simulink model "distances"  (R2018b)
settings: Solver=VariableStepAuto  StartTime=0.0  StopTime=1000  RelTol=1e-3
settings Model: Creator=User  LastModifiedBy=User

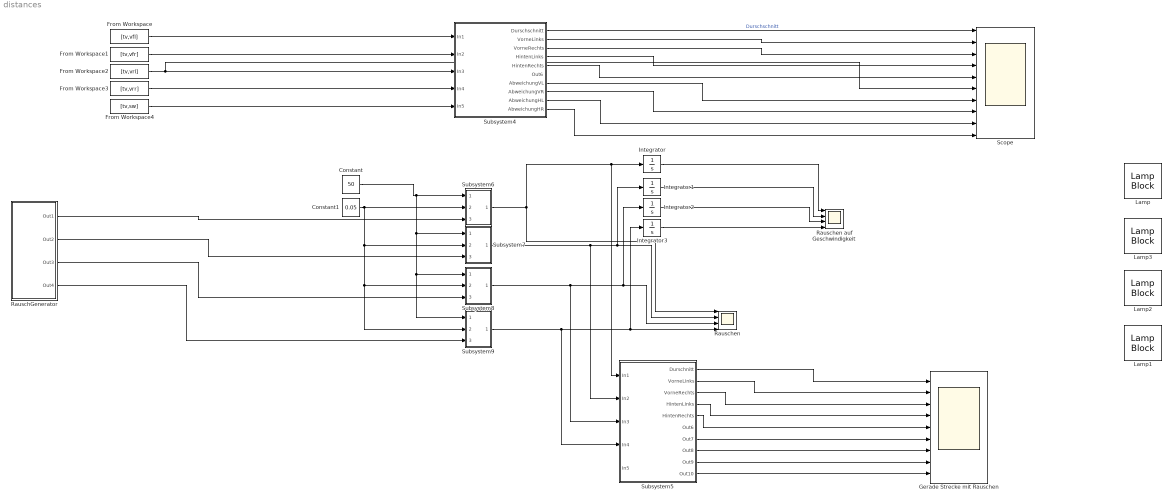
== system distances ==
  Constant : Constant  Value=50
  Constant1 : Constant  Value=0.05
  From Workspace : FromWorkspace  VariableName=[tv,vfl]
  From Workspace1 : FromWorkspace  VariableName=[tv,vfr]
  From Workspace2 : FromWorkspace  VariableName=[tv,vrl]
  From Workspace3 : FromWorkspace  VariableName=[tv,vrr]
  From Workspace4 : FromWorkspace  VariableName=[tv,sw]
  "Gerade Strecke mit Rauschen " : Scope  NumInputPorts=9
  Integrator{,1..3} (4 alike) : Integrator
  Lamp : LampBlock  WebBlockId=126
  Lamp1 : LampBlock  WebBlockId=127
  Lamp2 : LampBlock  WebBlockId=128
  Lamp3 : LampBlock  WebBlockId=129
  RauschGenerator : Subsystem
  "Rauschen " : Scope  NumInputPorts=4
  "Rauschen auf Geschwindigkeit " : Scope  NumInputPorts=4
  Scope : Scope  NumInputPorts=10
  Subsystem4 : Subsystem
  Subsystem5 : Subsystem
  Subsystem6 : Subsystem
  Subsystem7 : Subsystem
  Subsystem8 : Subsystem
  Subsystem9 : Subsystem
  wires:
  From Workspace2/1 -> Subsystem4/3(In3), Scope/6
  From Workspace/1 -> Subsystem4/1(In1)
  From Workspace1/1 -> Subsystem4/2(In2)
  From Workspace3/1 -> Subsystem4/4(In4)
  From Workspace4/1 -> Subsystem4/5(In5)
  Subsystem4/1("Durschschnitt ") -> Scope/1  "Durschschnitt"
  Subsystem4/2(VorneLinks) -> Scope/2
  Subsystem4/3(VorneRechts) -> Scope/3
  Subsystem4/4(HintenLinks) -> Scope/4
  Subsystem4/5(HintenRechts) -> Scope/5
  Subsystem4/7(AbweichungVL) -> Scope/7
  Subsystem4/8(AbweichungVR) -> Scope/8
  Subsystem4/9(AbweichungHL) -> Scope/9
  Subsystem4/10("AbweichungHR ") -> Scope/10
  Subsystem5/2(VorneLinks) -> "Gerade Strecke mit Rauschen "/2
  Constant/1 -> Subsystem9/1(In1), Subsystem8/1(In1), Subsystem7/1(In1), Subsystem6/1(In1)
  Constant1/1 -> Subsystem9/2(In2), Subsystem8/2(In2), Subsystem7/2(In2), Subsystem6/2(In2)
  Subsystem6/1(Out1) -> "Rauschen "/1, Integrator/1, Subsystem5/1(In1)
  Subsystem7/1(Out1) -> "Rauschen "/2, Integrator1/1, Subsystem5/2(In2)
  Subsystem5/3(VorneRechts) -> "Gerade Strecke mit Rauschen "/3
  Subsystem5/4(HintenLinks) -> "Gerade Strecke mit Rauschen "/4
  Subsystem5/5(HintenRechts) -> "Gerade Strecke mit Rauschen "/5
  Integrator/1 -> "Rauschen auf Geschwindigkeit "/1
  Integrator1/1 -> "Rauschen auf Geschwindigkeit "/2
  Subsystem8/1(Out1) -> "Rauschen "/3, Integrator2/1, Subsystem5/3(In3)
  Integrator2/1 -> "Rauschen auf Geschwindigkeit "/3
  Integrator3/1 -> "Rauschen auf Geschwindigkeit "/4
  Subsystem9/1(Out1) -> "Rauschen "/4, Integrator3/1, Subsystem5/4(In4)
  RauschGenerator/1(Out1) -> Subsystem6/3(In3)
  RauschGenerator/2(Out2) -> Subsystem7/3(In3)
  RauschGenerator/3(Out3) -> Subsystem8/3(In3)
  RauschGenerator/4(Out4) -> Subsystem9/3(In3)
  Subsystem5/1(Durschnitt) -> "Gerade Strecke mit Rauschen "/1
  Subsystem5/7(Out7) -> "Gerade Strecke mit Rauschen "/6
  Subsystem5/8(Out8) -> "Gerade Strecke mit Rauschen "/7
  Subsystem5/9(Out9) -> "Gerade Strecke mit Rauschen "/8
  Subsystem5/10(Out10) -> "Gerade Strecke mit Rauschen "/9

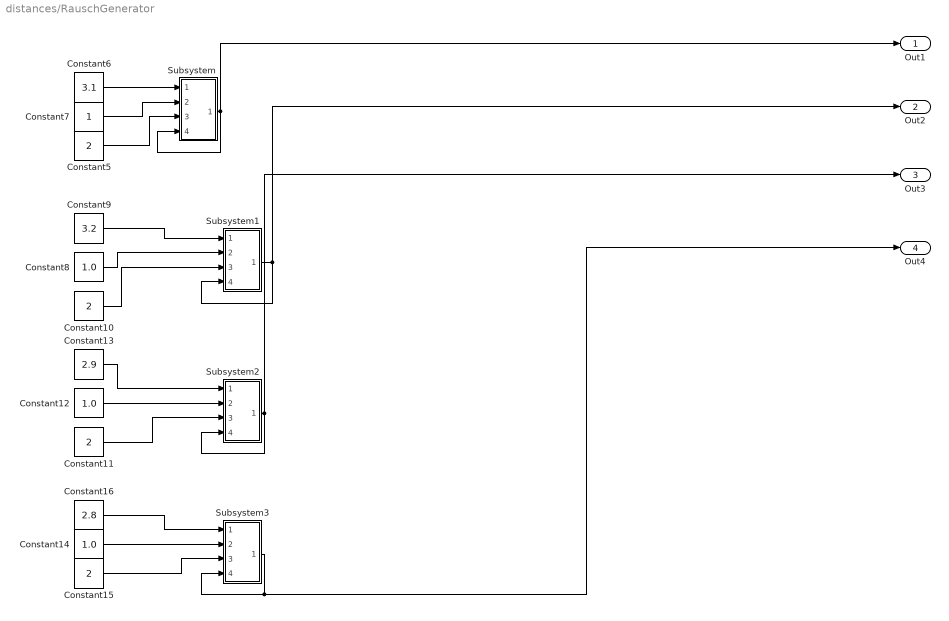
== system distances/RauschGenerator ==
  Constant{5,10..11,15} (4 alike) : Constant  Value=2
  Constant12 : Constant  Value=1.0
  Constant13 : Constant  Value=2.9
  Constant14 : Constant  Value=1.0
  Constant16 : Constant  Value=2.8
  Constant6 : Constant  Value=3.1
  Constant7 : Constant
  Constant8 : Constant  Value=1.0
  Constant9 : Constant  Value=3.2
  Subsystem : Subsystem
  Subsystem1 : Subsystem
  Subsystem2 : Subsystem
  Subsystem3 : Subsystem
  Out1 : Outport
  Out2 : Outport  Port=2
  Out3 : Outport  Port=3
  Out4 : Outport  Port=4
  wires:
  Constant16/1 -> Subsystem3/1(In1)
  Subsystem/1(Out1) -> Out1/1, Subsystem/4(In4)
  Constant11/1 -> Subsystem2/3(In3)
  Constant6/1 -> Subsystem/1(In1)
  Subsystem1/1(Out2) -> Out2/1, Subsystem1/4(In4)
  Subsystem3/1(Out1) -> Out4/1, Subsystem3/4(In4)
  Constant12/1 -> Subsystem2/2(In2)
  Constant5/1 -> Subsystem/3(In3)
  Subsystem2/1(Out1) -> Subsystem2/4(In4), Out3/1
  Constant10/1 -> Subsystem1/3(In3)
  Constant8/1 -> Subsystem1/2(In2)
  Constant9/1 -> Subsystem1/1(In1)
  Constant13/1 -> Subsystem2/1(In1)
  Constant15/1 -> Subsystem3/3(In3)
  Constant14/1 -> Subsystem3/2(In2)
  Constant7/1 -> Subsystem/2(In2)

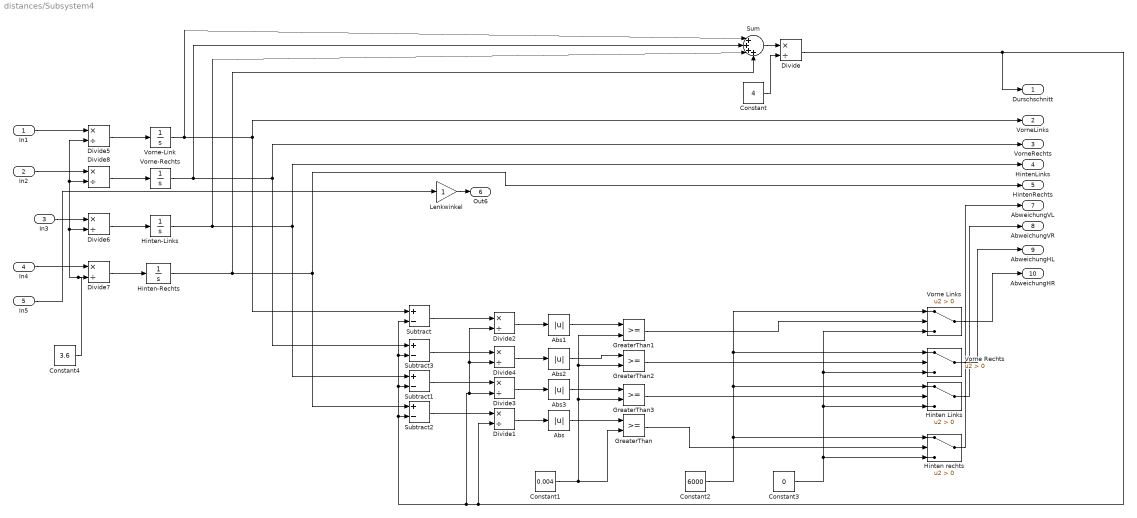
== system distances/Subsystem4 ==
  In1 : Inport
  In2 : Inport  Port=2
  In3 : Inport  Port=3
  In4 : Inport  Port=4
  In5 : Inport  Port=5
  Abs : Abs
  Abs1 : Abs  ZeroCross=off
  Abs2 : Abs
  Abs3 : Abs
  Constant : Constant  Value=4
  Constant1 : Constant  Value=0.004
  Constant2 : Constant  Value=6000
  Constant3 : Constant  Value=0
  Constant4 : Constant  Value=3.6
  Divide{,1..8} (9 alike) : Product  Inputs=*/
  GreaterThan{,1..3} (4 alike) : RelationalOperator  OutDataTypeStr=boolean  RndMeth=Simplest
  Hinten Links : Switch  Criteria=u2 > Threshold
  "Hinten rechts " : Switch  Criteria=u2 > Threshold
  Hinten-Links : Integrator  ContinuousStateAttributes='vfl'
  Hinten-Rechts : Integrator  ContinuousStateAttributes='vfl'
  Lenkwinkel : Gain
  Subtract{,1..3} (4 alike) : Sum  Inputs=+-
  Sum : Sum  Inputs=|++++
  "Vorne Links " : Switch  Criteria=u2 > Threshold
  "Vorne Rechts " : Switch  Criteria=u2 > Threshold
  Vorne-Link : Integrator  ContinuousStateAttributes='vfl'
  Vorne-Rechts : Integrator  ContinuousStateAttributes='vfl'
  "Durschschnitt " : Outport
  VorneLinks : Outport  Port=2
  VorneRechts : Outport  Port=3
  HintenLinks : Outport  Port=4
  HintenRechts : Outport  Port=5
  Out6 : Outport  Port=6
  AbweichungVL : Outport  Port=7
  AbweichungVR : Outport  Port=8
  AbweichungHL : Outport  Port=9
  "AbweichungHR " : Outport  Port=10
  wires:
  Divide5/1 -> Vorne-Link/1
  Divide/1 -> "Durschschnitt "/1, Subtract1/2, Subtract3/2, Subtract/2, Subtract2/2, Divide2/2, Divide4/2, Divide3/2, Divide1/2
  Vorne-Rechts/1 -> VorneRechts/1, Subtract3/1, Sum/2
  Constant4/1 -> Divide6/2, Divide8/2, Divide5/2, Divide7/2
  Abs2/1 -> GreaterThan2/1
  Constant/1 -> Divide/2
  Divide2/1 -> Abs1/1
  Constant3/1 -> "Vorne Links "/3, "Vorne Rechts "/3, Hinten Links/3, "Hinten rechts "/3
  Vorne-Link/1 -> Sum/1, VorneLinks/1, Subtract/1
  Constant2/1 -> "Vorne Links "/1, "Vorne Rechts "/1, Hinten Links/1, "Hinten rechts "/1
  GreaterThan/1 -> "Hinten rechts "/2
  Divide8/1 -> Vorne-Rechts/1
  Divide1/1 -> Abs/1
  Subtract2/1 -> Divide1/1
  Hinten-Links/1 -> HintenLinks/1, Subtract1/1, Sum/3
  Constant1/1 -> GreaterThan/2, GreaterThan3/2, GreaterThan2/2, GreaterThan1/2
  Divide6/1 -> Hinten-Links/1
  In1/1 -> Divide5/1
  Sum/1 -> Divide/1
  Abs3/1 -> GreaterThan3/1
  Abs1/1 -> GreaterThan1/1
  Hinten-Rechts/1 -> HintenRechts/1, Subtract2/1, Sum/4
  Subtract1/1 -> Divide3/1
  Divide4/1 -> Abs2/1
  GreaterThan1/1 -> "Vorne Links "/2
  Subtract/1 -> Divide2/1
  Abs/1 -> GreaterThan/1
  "Vorne Links "/1 -> "AbweichungHR "/1
  GreaterThan2/1 -> "Vorne Rechts "/2
  Subtract3/1 -> Divide4/1
  Divide7/1 -> Hinten-Rechts/1
  Divide3/1 -> Abs3/1
  GreaterThan3/1 -> Hinten Links/2
  "Hinten rechts "/1 -> AbweichungVL/1
  In2/1 -> Divide8/1
  "Vorne Rechts "/1 -> AbweichungHL/1
  In3/1 -> Divide6/1
  Hinten Links/1 -> AbweichungVR/1
  In5/1 -> Lenkwinkel/1
  Lenkwinkel/1 -> Out6/1
  In4/1 -> Divide7/1

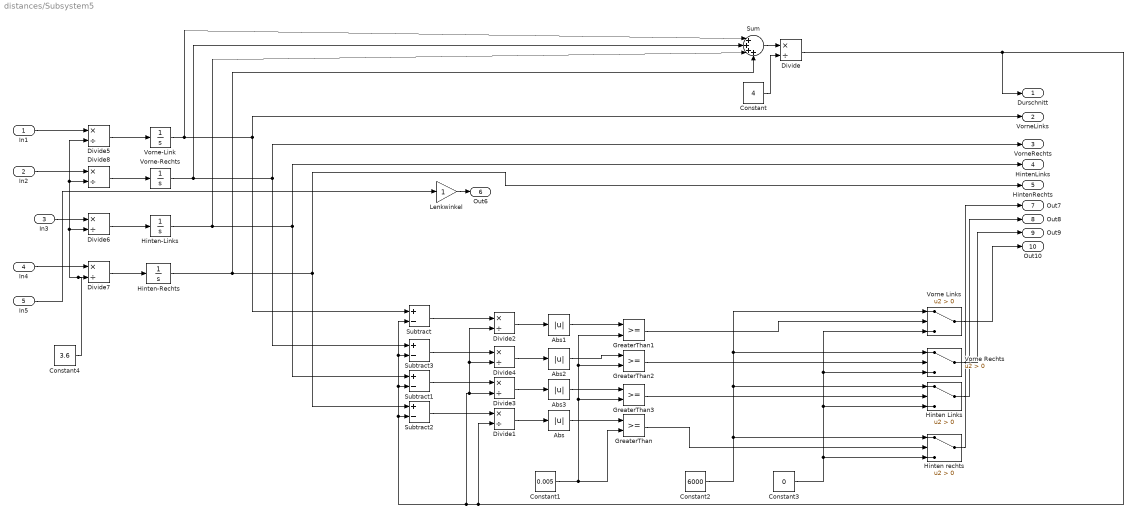
== system distances/Subsystem5 ==
  In1 : Inport
  In2 : Inport  Port=2
  In3 : Inport  Port=3
  In4 : Inport  Port=4
  In5 : Inport  Port=5
  Abs{,1..3} (4 alike) : Abs  ZeroCross=off
  Constant : Constant  Value=4
  Constant1 : Constant  Value=0.005
  Constant2 : Constant  Value=6000
  Constant3 : Constant  Value=0
  Constant4 : Constant  Value=3.6
  Divide{,1..8} (9 alike) : Product  Inputs=*/
  GreaterThan{,1..3} (4 alike) : RelationalOperator  OutDataTypeStr=boolean  ZeroCross=off  RndMeth=Simplest
  Hinten Links : Switch  Criteria=u2 > Threshold
  "Hinten rechts " : Switch  Criteria=u2 > Threshold
  Hinten-Links : Integrator  ContinuousStateAttributes='vfl'
  Hinten-Rechts : Integrator  ContinuousStateAttributes='vfl'
  Lenkwinkel : Gain
  Subtract{,1..3} (4 alike) : Sum  Inputs=+-
  Sum : Sum  Inputs=|++++
  "Vorne Links " : Switch  Criteria=u2 > Threshold
  "Vorne Rechts " : Switch  Criteria=u2 > Threshold
  Vorne-Link : Integrator  ContinuousStateAttributes='vfl'
  Vorne-Rechts : Integrator  ContinuousStateAttributes='vfl'
  Durschnitt : Outport
  VorneLinks : Outport  Port=2
  VorneRechts : Outport  Port=3
  HintenLinks : Outport  Port=4
  HintenRechts : Outport  Port=5
  Out6 : Outport  Port=6
  Out7 : Outport  Port=7
  Out8 : Outport  Port=8
  Out9 : Outport  Port=9
  Out10 : Outport  Port=10
  wires:
  Divide5/1 -> Vorne-Link/1
  Divide/1 -> Durschnitt/1, Subtract1/2, Subtract3/2, Subtract/2, Subtract2/2, Divide2/2, Divide4/2, Divide3/2, Divide1/2
  Vorne-Rechts/1 -> VorneRechts/1, Subtract3/1, Sum/2
  Constant4/1 -> Divide6/2, Divide8/2, Divide5/2, Divide7/2
  Abs2/1 -> GreaterThan2/1
  Constant/1 -> Divide/2
  Divide2/1 -> Abs1/1
  Constant3/1 -> "Vorne Links "/3, "Vorne Rechts "/3, Hinten Links/3, "Hinten rechts "/3
  Vorne-Link/1 -> Sum/1, VorneLinks/1, Subtract/1
  Constant2/1 -> "Vorne Links "/1, "Vorne Rechts "/1, Hinten Links/1, "Hinten rechts "/1
  GreaterThan/1 -> "Hinten rechts "/2
  Divide8/1 -> Vorne-Rechts/1
  Divide1/1 -> Abs/1
  Subtract2/1 -> Divide1/1
  Hinten-Links/1 -> HintenLinks/1, Subtract1/1, Sum/3
  Constant1/1 -> GreaterThan/2, GreaterThan3/2, GreaterThan2/2, GreaterThan1/2
  Divide6/1 -> Hinten-Links/1
  In1/1 -> Divide5/1
  Sum/1 -> Divide/1
  Abs3/1 -> GreaterThan3/1
  Abs1/1 -> GreaterThan1/1
  Hinten-Rechts/1 -> HintenRechts/1, Subtract2/1, Sum/4
  Subtract1/1 -> Divide3/1
  Divide4/1 -> Abs2/1
  GreaterThan1/1 -> "Vorne Links "/2
  Subtract/1 -> Divide2/1
  Abs/1 -> GreaterThan/1
  "Vorne Links "/1 -> Out10/1
  GreaterThan2/1 -> "Vorne Rechts "/2
  Subtract3/1 -> Divide4/1
  Divide7/1 -> Hinten-Rechts/1
  Divide3/1 -> Abs3/1
  GreaterThan3/1 -> Hinten Links/2
  "Hinten rechts "/1 -> Out7/1
  In2/1 -> Divide8/1
  "Vorne Rechts "/1 -> Out9/1
  In3/1 -> Divide6/1
  Hinten Links/1 -> Out8/1
  In5/1 -> Lenkwinkel/1
  Lenkwinkel/1 -> Out6/1
  In4/1 -> Divide7/1

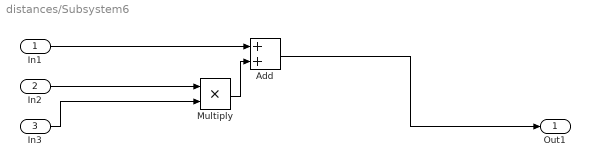
== system distances/Subsystem6 ==
  In1 : Inport
  In2 : Inport  Port=2
  In3 : Inport  Port=3
  Add : Sum
  Multiply : Product
  Out1 : Outport
  wires:
  Add/1 -> Out1/1
  Multiply/1 -> Add/2
  In3/1 -> Multiply/2
  In1/1 -> Add/1
  In2/1 -> Multiply/1

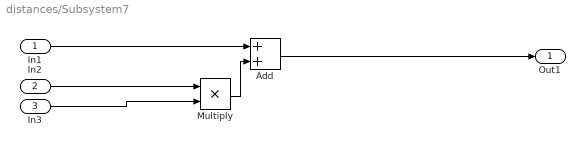
== system distances/Subsystem7 ==
  In1 : Inport
  In2 : Inport  Port=2
  In3 : Inport  Port=3
  Add : Sum
  Multiply : Product
  Out1 : Outport
  wires:
  Add/1 -> Out1/1
  Multiply/1 -> Add/2
  In3/1 -> Multiply/2
  In1/1 -> Add/1
  In2/1 -> Multiply/1

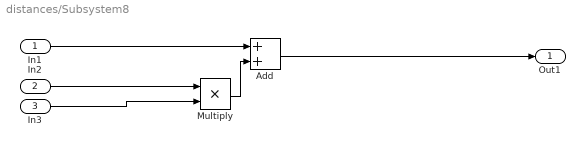
== system distances/Subsystem8 ==
  In1 : Inport
  In2 : Inport  Port=2
  In3 : Inport  Port=3
  Add : Sum
  Multiply : Product
  Out1 : Outport
  wires:
  Add/1 -> Out1/1
  Multiply/1 -> Add/2
  In3/1 -> Multiply/2
  In1/1 -> Add/1
  In2/1 -> Multiply/1

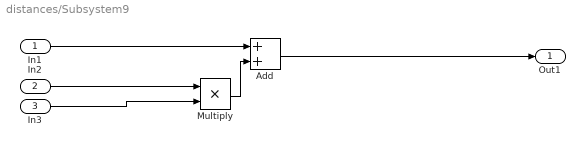
== system distances/Subsystem9 ==
  In1 : Inport
  In2 : Inport  Port=2
  In3 : Inport  Port=3
  Add : Sum
  Multiply : Product
  Out1 : Outport
  wires:
  Add/1 -> Out1/1
  Multiply/1 -> Add/2
  In3/1 -> Multiply/2
  In1/1 -> Add/1
  In2/1 -> Multiply/1

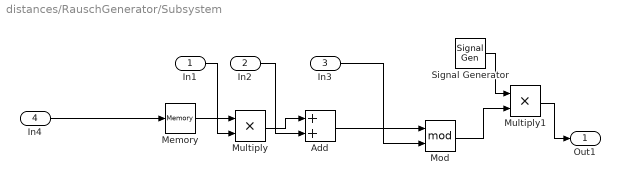
== system distances/RauschGenerator/Subsystem ==
  In1 : Inport
  In2 : Inport  Port=2
  In3 : Inport  Port=3
  In4 : Inport  Port=4
  Add : Sum
  Memory : Memory  InitialCondition=1
  Mod : Math  Operator=mod  SaturateOnIntegerOverflow=on
  Multiply : Product
  Multiply1 : Product
  Signal Generator : SignalGenerator  Units=rad/sec
  Out1 : Outport
  wires:
  In3/1 -> Mod/2
  Multiply/1 -> Add/1
  Memory/1 -> Multiply/1
  Mod/1 -> Multiply1/2
  Add/1 -> Mod/1
  In2/1 -> Add/2
  In4/1 -> Memory/1
  In1/1 -> Multiply/2
  Multiply1/1 -> Out1/1
  Signal Generator/1 -> Multiply1/1

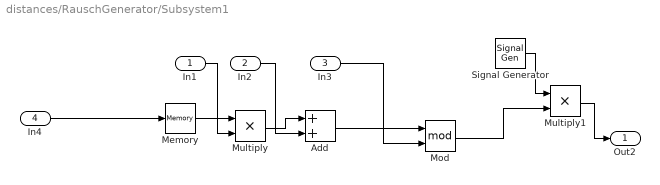
== system distances/RauschGenerator/Subsystem1 ==
  In1 : Inport
  In2 : Inport  Port=2
  In3 : Inport  Port=3
  In4 : Inport  Port=4
  Add : Sum
  Memory : Memory  InitialCondition=1
  Mod : Math  Operator=mod  SaturateOnIntegerOverflow=on
  Multiply : Product
  Multiply1 : Product
  Signal Generator : SignalGenerator  Units=rad/sec
  Out2 : Outport
  wires:
  In3/1 -> Mod/2
  Multiply/1 -> Add/1
  Memory/1 -> Multiply/1
  Add/1 -> Mod/1
  In2/1 -> Add/2
  In4/1 -> Memory/1
  In1/1 -> Multiply/2
  Signal Generator/1 -> Multiply1/1
  Multiply1/1 -> Out2/1
  Mod/1 -> Multiply1/2

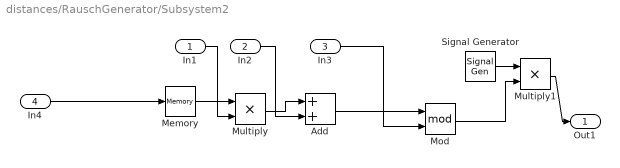
== system distances/RauschGenerator/Subsystem2 ==
  In1 : Inport
  In2 : Inport  Port=2
  In3 : Inport  Port=3
  In4 : Inport  Port=4
  Add : Sum
  Memory : Memory  InitialCondition=1
  Mod : Math  Operator=mod  SaturateOnIntegerOverflow=on
  Multiply : Product
  Multiply1 : Product
  Signal Generator : SignalGenerator  Units=rad/sec
  Out1 : Outport
  wires:
  In3/1 -> Mod/2
  Multiply/1 -> Add/1
  Memory/1 -> Multiply/1
  Mod/1 -> Multiply1/2
  Add/1 -> Mod/1
  In2/1 -> Add/2
  In4/1 -> Memory/1
  In1/1 -> Multiply/2
  Signal Generator/1 -> Multiply1/1
  Multiply1/1 -> Out1/1

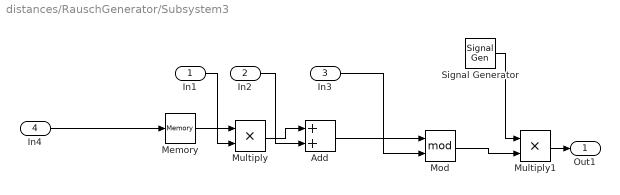
== system distances/RauschGenerator/Subsystem3 ==
  In1 : Inport
  In2 : Inport  Port=2
  In3 : Inport  Port=3
  In4 : Inport  Port=4
  Add : Sum
  Memory : Memory  InitialCondition=1
  Mod : Math  Operator=mod  SaturateOnIntegerOverflow=on
  Multiply : Product
  Multiply1 : Product
  Signal Generator : SignalGenerator  Units=rad/sec
  Out1 : Outport
  wires:
  In3/1 -> Mod/2
  Multiply/1 -> Add/1
  Memory/1 -> Multiply/1
  Mod/1 -> Multiply1/2
  Add/1 -> Mod/1
  In2/1 -> Add/2
  In4/1 -> Memory/1
  In1/1 -> Multiply/2
  Signal Generator/1 -> Multiply1/1
  Multiply1/1 -> Out1/1
